simulink model "test_pid_tv"  (R2024b)
settings: Solver=VariableStepAuto  StartTime=0.0  StopTime=10.0  RelTol=1e-3
model workspace (MAT data in the model file):
  Sig = Simulink.Signal
  Sig.Dimensions = -1
  Sig.DimensionsMode = 'auto'
  Sig.Complexity = 'auto'
  Sig.SampleTime = -1
  Sig.SamplingMode = 'auto'
  Sig.DataType = 'auto'
  mbd_rack_movement = [-24.295 -24.2949831878 -24.2949831878 -24.2949831878 -24.2949831877 -24.2949831876 -24.2949831874 -24.2949831869 -24.2949831849 -24.2949831786 -24.2949831545 -24.2949831492 ... (273 elements, 273x1)]
  rack_mm = [-25.136 -25.1276327886 -25.1095284284 -25.0914240682 -25.073319708 -25.0564044471 -25.0415413809 -25.0266783147 -25.0118152486 -24.9987131808 -24.9886873592 -24.9786615375 ... (4070 elements, 4070x1)]
  steer_sensor = [701.530379071 702.453261845 703.675449618 704.897637391 706.119825165 707.135081137 707.617795373 708.10050961 708.583223846 709.091528196 709.761580489 710.431632781 ... (4070 elements, 4070x1)]
  wheel_steer_left = [22.9038666573 22.9079555 22.904490995 22.7859585761 22.785958576 22.7859585758 22.7859585755 22.7859585748 22.7859585724 22.7859585657 22.7859585412 22.7859585359 ... (273 elements, 273x1)]
  wheel_steer_right = [23.2682364009 23.2679586767 23.2681940775 23.3035254873 23.3035254873 23.3035254872 23.3035254871 23.3035254866 23.3035254847 23.3035254783 23.3035254538 23.3035254484 ... (273 elements, 273x1)]
libraries: simulink_extras x1, slpidlib x1
settings Model: Creator=lukec  LastModifiedBy=ben

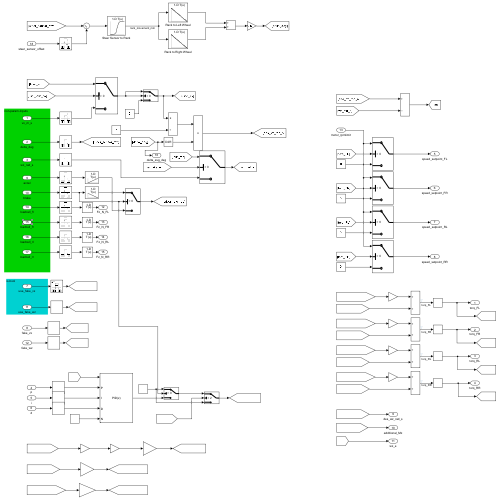
[thumbnail: Simulink's stored preview of the top-level diagram]
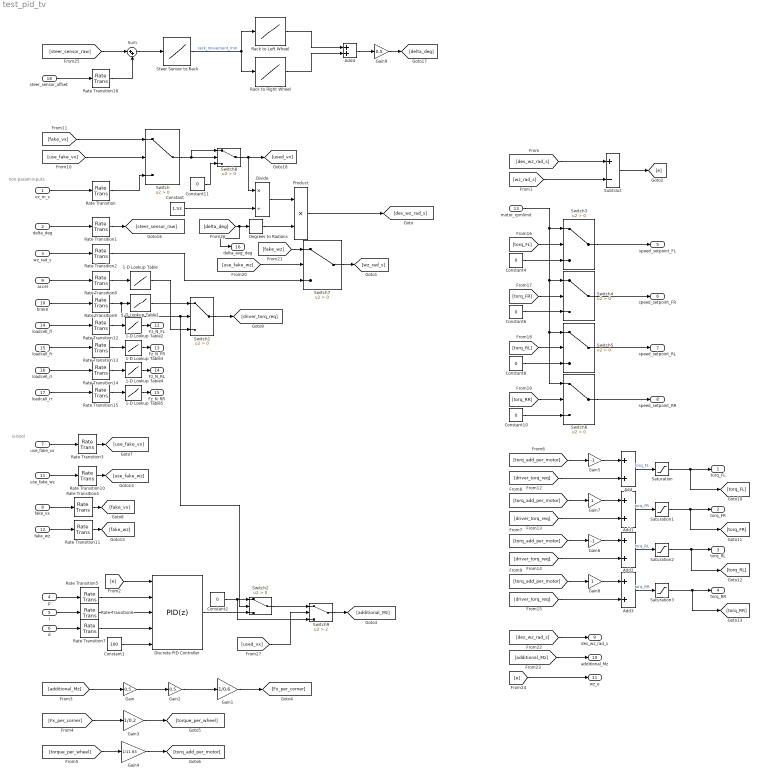
== system test_pid_tv ==
  note: non-param-inputs
  note: is-bool
  vx_m_s : Inport
  delta_deg : Inport  Port=2
  wz_rad_s : Inport  Port=3
  p : Inport  Port=4
  i : Inport  Port=5
  d : Inport  Port=6
  use_fake_vx : Inport  Port=7
  fake_vx : Inport  Port=8
  accel : Inport  Port=9
  brake : Inport  Port=10
  use_fake_wz : Inport  Port=11
  fake_wz : Inport  Port=12
  motor_rpmlimit : Inport  Port=13
  loadcell_fl : Inport  Port=14
  loadcell_fr : Inport  Port=15
  loadcell_rl : Inport  Port=16
  loadcell_rr : Inport  Port=17
  steer_sensor_offset : Inport  Port=18
  1-D Lookup Table : Lookup_n-D  NumberOfTableDimensions=1  BreakpointsForDimension1=[0 1]  Table=[0 21]  InternalRulePriority=Speed  RndMeth=Simplest
  1-D Lookup Table1 : Lookup_n-D  NumberOfTableDimensions=1  BreakpointsForDimension1=[0 1]  Table=[0 -21]  InternalRulePriority=Speed  RndMeth=Simplest
  1-D Lookup Table2 : Lookup_n-D  NumberOfTableDimensions=1  BreakpointsForDimension1=[0 71 227 264 464 569 704 797 909 1076 1234]  Table=[0 11.8 22.2 37.5 63.2 79 102.1 120.3 133 154 174].*4.448  InternalRulePriority=Speed  RndMeth=Simplest
  1-D Lookup Table3 : Lookup_n-D  NumberOfTableDimensions=1  BreakpointsForDimension1=[0 6 207 312 449 547 666 709 803 969]  Table=[0 31.1 57.9 74.4 100.3 117 129.5 134 143 167.8].*4.448  InternalRulePriority=Speed  RndMeth=Simplest
  1-D Lookup Table4 : Lookup_n-D  NumberOfTableDimensions=1  BreakpointsForDimension1=[0 122 148 266 351 429 511 565 661 767 900 1023]  Table=[0 28.1 33 50.6 64.7 81 96.4 107.3 123.2 139.5 160.5 180.5].*4.448  InternalRulePriority=Speed  RndMeth=Simplest
  1-D Lookup Table5 : Lookup_n-D  NumberOfTableDimensions=1  BreakpointsForDimension1=[0 110 158 273 355 435 512 589 677 785 906 996]  Table=[0 27.6 35.8 52.9 67 83.6 98.3 109.2 125.9 142.9 160 175.2].*4.448  InternalRulePriority=Speed  RndMeth=Simplest
  Add{,1..4} (5 alike) : Sum
  Constant : Constant  Value=1.53
  Constant1 : Constant  Value=100
  Constant{2,4,6,8,10..11} (6 alike) : Constant  Value=0
  Degrees to Radians : simulink_extras/Transformations/Degrees to Radians
  Discrete PID Controller : slpidlib/PID Controller  Controller=PID  Form=Parallel  TimeDomain=Discrete-time  UseExternalTs=off  SampleTime=-1  IntegratorMethod=Forward Euler  FilterMethod=Forward Euler  ControllerParametersSource=external  P=1  I=1  UseKiTs=off  D=0  UseExternalDerivativeSource=off  N=100  UseFilter=on  TunerSelectOption=Transfer Function Based (PID Tuner App)  InitialConditionSource=internal  InitialConditionForIntegrator=0  InitialConditionForFilter=0  DifferentiatorICPrevScaledInput=0  ExternalReset=none  TrackingMode=off  Kt=1  LimitOutput=off  SatLimitsSource=internal  UpperSaturationLimit=inf  LowerSaturationLimit=-inf  LinearizeAsGain=off  AntiWindupMode=none  Kb=1  LimitIntegrator=off  UpperIntegratorSaturationLimit=inf  LowerIntegratorSaturationLimit=-inf  POutMin=[]  POutMax=[]  IOutMin=[]  IOutMax=[]  DOutMin=[]  DOutMax=[]  NOutMin=[]  NOutMax=[]  SumOutMin=[]  SumOutMax=[]  SaturationOutMin=[]  SaturationOutMax=[]  PParamMin=[]  PParamMax=[]  IParamMin=[]  IParamMax=[]  DParamMin=[]  DParamMax=[]  NParamMin=[]  NParamMax=[]  KbParamMin=[]  KbParamMax=[]  KtParamMin=[]  KtParamMax=[]  KbOutMin=[]  KbOutMax=[]  KtOutMin=[]  KtOutMax=[]  IntegratorOutMin=[]  IntegratorOutMax=[]  FilterOutMin=[]  FilterOutMax=[]  SumI1OutMin=[]  SumI1OutMax=[]  SumI2OutMin=[]  SumI2OutMax=[]  SumI3OutMin=[]  SumI3OutMax=[]  SumI4OutMin=[]  SumI4OutMax=[]  SumDOutMin=[]  SumDOutMax=[]  DifferentiatorOutMin=[]  DifferentiatorOutMax=[]  FilterDiffOutCoefMin=[]  FilterDiffOutCoefMax=[]  ReciprocalOutMin=[]  ReciprocalOutMax=[]  SumDenOutMin=[]  SumDenOutMax=[]  SumNumOutMin=[]  SumNumOutMax=[]  DivideOutMin=[]  DivideOutMax=[]  UdiffTsProdOutMin=[]  UdiffTsProdOutMax=[]  NTsProdOutMin=[]  NTsProdOutMax=[]  UintegralTsProdOutMin=[]  UintegralTsProdOutMax=[]  UngainTsProdOutMin=[]  UngainTsProdOutMax=[]  ClampingZeroOutDataTypeStr=Inherit: Inherit via back propagation  ClampingZeroOutMin=[]  ClampingZeroOutMax=[]  FilterDenConstantOutDataTypeStr=Inherit: Inherit via back propagation  FilterDenConstantOutMin=[]  FilterDenConstantOutMax=[]  PCopyOutDataTypeStr=Inherit: Inherit via back propagation  PCopyOutMin=[]  PCopyOutMax=[]  NCopyOutDataTypeStr=Inherit: Inherit via back propagation  NCopyOutMin=[]  NCopyOutMax=[]  IntegratorContinuousStateAttributes=''  IntegratorStateMustResolveToSignalObject=off  IntegratorRTWStateStorageClass=Auto  FilterContinuousStateAttributes=''  FilterStateMustResolveToSignalObject=off  FilterRTWStateStorageClass=Auto  ParallelPVariant=ExternalParameters  IdealPVariant=Disabled  IVariant=ExternalParameters  DVariant=ExternalParameters  IntegratorVariant=Discrete  SatVariant=Disabled  AWVariant=Passthrough  PCopyVariant=Disabled  TRVariant=Disabled  FdbkBlocksVariant=Forward  IdealPFdbkVariant=Disabled  SatFdbkVariant=Disabled  DerivativeFilterVariant=ForwardEulerFilter  NVariant=ExternalParameters  NCopyVariant=Disabled  FilterICVariant=InternalICsFilter  IntegratorICVariant=InternalICs  ExternalResetVariant=Disabled  TRSumVariant=Passthrough  SumFdbkVariant=Disabled  SumVariant=Sum_PID  TsampFilterVariant=InternalTs  TsampNgainVariant=Passthrough  TsampIntegralVariant=Disabled_SignalSpec  ExternalSaturationOutDataTypeStr=Inherit: Same as second input  DerivativeSourceVariant=ErrorSignal  PreIntVariant=InternalPreInt
      settings: LibrarySourceBlock=simulink/Discrete/Discrete PID Controller
  Divide : Product  Inputs=*/
  Gain : Gain  Gain=0.5
  Gain1 : Gain  Gain=1/0.6
  Gain2 : Gain  Gain=0.5
  Gain3 : Gain  Gain=1/0.2
  Gain4 : Gain  Gain=1/11.83
  Gain5 : Gain  Gain=-1
  Gain6 : Gain  Gain=-1
  Gain7 : Gain
  Gain8 : Gain
  Gain9 : Gain  Gain=0.5
  Product : Product
  Rack to Left Wheel : Lookup_n-D  NumberOfTableDimensions=1  BreakpointsForDimension1=mbd_rack_movement  Table=wheel_steer_left  ExtrapMethod=Clip  UseLastTableValue=on  InternalRulePriority=Speed  RndMeth=Simplest
  Rack to Right Wheel : Lookup_n-D  NumberOfTableDimensions=1  BreakpointsForDimension1=mbd_rack_movement  Table=wheel_steer_right  ExtrapMethod=Clip  UseLastTableValue=on  InternalRulePriority=Speed  RndMeth=Simplest
  Rate Transition{,1..16} (17 alike) : RateTransition  OutPortSampleTime=0.01
  Saturation{,1..3} (4 alike) : Saturate  UpperLimit=21  LowerLimit=-21
  Steer Sensor to Rack : Lookup_n-D  NumberOfTableDimensions=1  LookupTableObject=PLEASE  BreakpointsForDimension1=steer_sensor  Table=rack_mm  ExtrapMethod=Clip  InternalRulePriority=Speed  RndMeth=Simplest
  Subtract : Sum  Inputs=+-
  Sum : Sum  Inputs=|++
  Switch{,1..8} (9 alike) : Switch  Criteria=u2 > Threshold  SaturateOnIntegerOverflow=off  InputSameDT=off
  Switch9 : Switch  Criteria=u2 > Threshold  Threshold=2  SaturateOnIntegerOverflow=off  InputSameDT=off
  torq_FL : Outport
  torq_FR : Outport  Port=2
  torq_RL : Outport  Port=3
  torq_RR : Outport  Port=4
  speed_setpoint_FL : Outport  Port=5
  speed_setpoint_FR : Outport  Port=6
  speed_setpoint_RL : Outport  Port=7
  speed_setpoint_RR : Outport  Port=8
  des_wz_rad_s : Outport  Port=9
  additional_Mz : Outport  Port=10
  wz_e : Outport  Port=11
  Fz_N_FL : Outport  Port=12
  Fz_N_FR : Outport  Port=13
  Fz_N_RL : Outport  Port=14
  Fz_N_RR : Outport  Port=15
  delta_avg_deg : Outport  Port=16
  wires:
  Constant/1 -> Divide/2
  Divide/1 -> Product/1
  delta_deg/1 -> Rate Transition1/1
  [des_wz_rad_s] -> Subtract/1
  wz_rad_s/1 -> Rate Transition2/1
  [wz_rad_s] -> Subtract/2
  Subtract/1 -> [e]
  [e] -> Discrete PID Controller/1
  p/1 -> Rate Transition5/1
  i/1 -> Rate Transition6/1
  d/1 -> Rate Transition7/1
  Constant1/1 -> Discrete PID Controller/5
  [additional_Mz] -> Gain/1
  Gain/1 -> Gain2/1
  Gain2/1 -> Gain1/1
  Gain1/1 -> [Fx_per_corner]
  [Fx_per_corner] -> Gain3/1
  Gain3/1 -> [torque_per_wheel]
  [torque_per_wheel] -> Gain4/1
  Gain4/1 -> [torq_add_per_motor]
  [torq_add_per_motor] -> Gain5/1
  [torq_add_per_motor] -> Gain6/1
  [torq_add_per_motor] -> Gain7/1
  [torq_add_per_motor] -> Gain8/1
  use_fake_vx/1 -> Rate Transition3/1
  fake_vx/1 -> Rate Transition4/1
  [use_fake_vx] -> Switch/2
  [fake_vx] -> Switch/1
  vx_m_s/1 -> Rate Transition/1
  Rate Transition/1 -> Switch/3
  Rate Transition1/1 -> [steer_sensor_raw]
  Rate Transition3/1 -> [use_fake_vx]
  Rate Transition4/1 -> [fake_vx]
  Rate Transition5/1 -> Discrete PID Controller/2
  Rate Transition6/1 -> Discrete PID Controller/3
  Rate Transition7/1 -> Discrete PID Controller/4
  accel/1 -> Rate Transition8/1
  brake/1 -> Rate Transition9/1
  Rate Transition8/1 -> 1-D Lookup Table/1
  Rate Transition9/1 -> Switch2/2, Switch1/2, 1-D Lookup Table1/1
  Switch1/1 -> [driver_torq_req]
  Gain5/1 -> Add/1
  Add/1 -> Saturation/1  "torq_FL"
  1-D Lookup Table1/1 -> Switch1/1
  1-D Lookup Table/1 -> Switch1/3
  [driver_torq_req] -> Add/2
  [driver_torq_req] -> Add1/2
  Add1/1 -> Saturation1/1  "torq_FR"
  Gain7/1 -> Add1/1
  Gain6/1 -> Add2/1
  Add2/1 -> Saturation2/1  "torq_RL"
  Add3/1 -> Saturation3/1  "torq_RR"
  Gain8/1 -> Add3/1
  [driver_torq_req] -> Add2/2
  [driver_torq_req] -> Add3/2
  Discrete PID Controller/1 -> Switch2/3
  Constant2/1 -> Switch9/3, Switch2/1
  Constant4/1 -> Switch3/3
  Switch3/1 -> speed_setpoint_FL/1
  [torq_FL] -> Switch3/2
  [torq_FR] -> Switch4/2
  Constant6/1 -> Switch4/3
  Constant8/1 -> Switch5/3
  [torq_RL] -> Switch5/2
  [torq_RR] -> Switch6/2
  Constant10/1 -> Switch6/3
  Switch6/1 -> speed_setpoint_RR/1
  Switch5/1 -> speed_setpoint_RL/1
  Switch4/1 -> speed_setpoint_FR/1
  use_fake_wz/1 -> Rate Transition10/1
  Rate Transition10/1 -> [use_fake_wz]
  fake_wz/1 -> Rate Transition11/1
  Rate Transition11/1 -> [fake_wz]
  [use_fake_wz] -> Switch7/2
  [fake_wz] -> Switch7/1
  Switch7/1 -> [wz_rad_s]
  Rate Transition2/1 -> Switch7/3
  [des_wz_rad_s] -> des_wz_rad_s/1
  [additional_Mz] -> additional_Mz/1
  [e] -> wz_e/1
  Saturation/1 -> [torq_FL], torq_FL/1
  Saturation1/1 -> [torq_FR], torq_FR/1
  Saturation2/1 -> [torq_RL], torq_RL/1
  Saturation3/1 -> [torq_RR], torq_RR/1
  Switch/1 -> Switch8/1, Switch8/2
  Switch8/1 -> Divide/1, [used_vx]
  Constant11/1 -> Switch8/3
  motor_rpmlimit/1 -> Switch6/1, Switch5/1, Switch4/1, Switch3/1
  Rack to Left Wheel/1 -> Add4/1
  Steer Sensor to Rack/1 -> Rack to Left Wheel/1, Rack to Right Wheel/1  "rack_movement_mm"
  Rack to Right Wheel/1 -> Add4/2
  Add4/1 -> Gain9/1
  Gain9/1 -> [delta_deg]
  Degrees to Radians/1 -> Product/2
  [delta_deg] -> delta_avg_deg/1, Degrees to Radians/1
  Product/1 -> [des_wz_rad_s]
  Switch9/1 -> [additional_Mz]
  Switch2/1 -> Switch9/1
  [used_vx] -> Switch9/2
  loadcell_fl/1 -> Rate Transition12/1
  loadcell_fr/1 -> Rate Transition13/1
  loadcell_rl/1 -> Rate Transition14/1
  loadcell_rr/1 -> Rate Transition15/1
  Rate Transition12/1 -> 1-D Lookup Table2/1
  Rate Transition13/1 -> 1-D Lookup Table3/1
  Rate Transition14/1 -> 1-D Lookup Table4/1
  Rate Transition15/1 -> 1-D Lookup Table5/1
  1-D Lookup Table2/1 -> Fz_N_FL/1
  1-D Lookup Table3/1 -> Fz_N_FR/1
  1-D Lookup Table4/1 -> Fz_N_RL/1
  1-D Lookup Table5/1 -> Fz_N_RR/1
  [steer_sensor_raw] -> Sum/1
  Sum/1 -> Steer Sensor to Rack/1
  steer_sensor_offset/1 -> Rate Transition16/1
  Rate Transition16/1 -> Sum/2
